simulink model "s_dbip"  (Simulink 7.7)
settings: Solver=ode1  StartTime=0.0  StopTime=100  FixedStep=0.001  RelTol=1e-3
values from neighbouring files (symbols this model uses):
  A = [0 0 0 1 0 0 ... (first row only)    [DBIP_ABCD_eqns.m]
  B = Kg * kt * B / Rm    [DBIP_ABCD_eqns.m]    (also in Symbolic_EL_Calculations.m = [1;0])
  C = eye(6,6)    [DBIP_ABCD_eqns.m]    (also in Symbolic_EL_Calculations.m = [0 theta2dot*sin(theta1 - theta2))
  D = zeros(6,1)    [DBIP_ABCD_eqns.m]
  X0 = [-5, 1, -0.5, 0, 0, 0] * pi / 180    [setup_dbip.m]
undefined symbols (not defined in the file or in its folder): k
libraries: simulink_extras x5
settings Model: Creator=MLevis  LastModifiedBy=MLevis  ExtModeTrigDuration=10000  ExtModeArmWhenConnect=off  BufferReuse=off
settings SolverCC: PositivePriorityOrder=on
settings OptimizationCC: BooleanDataType=off  InlineInvariantSignals=on  OptimizeBlockIOStorage=off  BufferReuse=off  ExpressionFolding=off  LocalBlockOutputs=off  InitFltsAndDblsToZero=on
settings DebuggingCC: SaveWithParameterizedLinksMsg=none  SignalResolutionControl=TryResolveAllWithWarning  SolverPrmCheckMsg=none  MultiTaskDSMMsg=warning  MultiTaskCondExecSysMsg=none  StrictBusMsg=None
settings RTWCC: SystemTargetFile=quarc_windows.tlc  TemplateMakefile=quarc_default_tmf  Description=QuaRC Win32 Target  ProcessScript=quarc_windows_make_rtw_hook  IncludeERTFirstTime=on
settings STFCustomTargetCC: TargetFcnLib=ansi_tfl_tmw.mat  TargetPreCompLibLocation=C:\PROGRA~3\QUARC\lib\2011a\windows\release  FunctionExecutionProfile=off  GeneratePreprocessorConditionals=Disable all  SystemTargetFile=quarc_windows.tlc
settings GRTTargetCC: TargetFcnLib=ansi_tfl_tmw.mat  TargetPreCompLibLocation=C:\PROGRA~3\QUARC\lib\2011a\windows\release  ParMdlRefBuildCompliant=off  CompOptLevelCompliant=off  MatFileLogging=off  ExtMode=on  ExtModeMexFile=quarc_comm

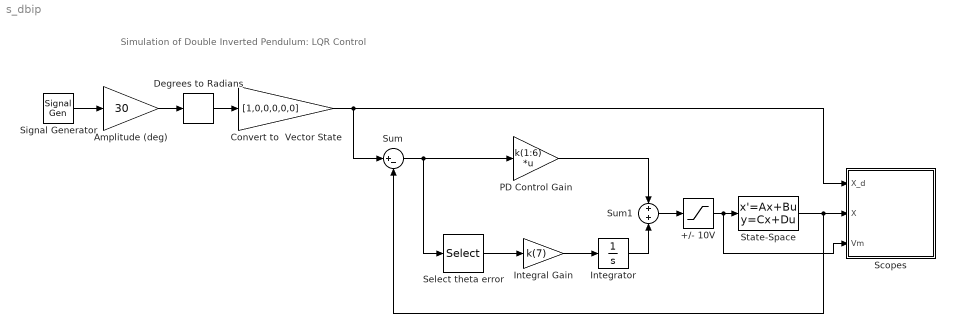
== system s_dbip ==
  note: Simulation of Double Inverted Pendulum: LQR Control
  +/- 10V : Saturate  UpperLimit=10  LowerLimit=-10
  Amplitude (deg) : Gain  Gain=30  SaturateOnIntegerOverflow=on  OutDataTypeStr=Inherit: Same as input  ParamDataTypeStr=Inherit: Same as input
  Convert to  Vector State : Gain  Gain=[1,0,0,0,0,0]
  Degrees to Radians : simulink_extras/Transformations/Degrees to Radians  SystemSampleTime=-1
  Integral Gain : Gain  Gain=k(7)
  Integrator : Integrator
  PD Control Gain : Gain  Gain=k(1:6)  Multiplication=Matrix(K*u)  SaturateOnIntegerOverflow=on  OutDataTypeStr=Inherit: Same as input  ParamDataTypeStr=Inherit: Same as input
  Scopes : Subsystem
  Select theta error : Selector  InputPortWidth=6  IndexOptions=Index vector (dialog)  Indices=1  OutputSizes=1
  Signal Generator : SignalGenerator  WaveForm=square  Frequency=0.02
  State-Space : StateSpace  A=A  B=B  C=C  D=D  X0=X0
  Sum : Sum  Inputs=|+-
  Sum1 : Sum
  wires:
  Signal Generator/1 -> Amplitude (deg)/1
  Amplitude (deg)/1 -> Degrees to Radians/1
  Degrees to Radians/1 -> Convert to  Vector State/1
  Convert to  Vector State/1 -> Sum/1, Scopes/1(X_d)
  Sum/1 -> PD Control Gain/1, Select theta error/1
  Sum1/1 -> +/- 10V/1
  Integral Gain/1 -> Integrator/1
  Select theta error/1 -> Integral Gain/1
  Integrator/1 -> Sum1/2
  PD Control Gain/1 -> Sum1/1
  State-Space/1 -> Scopes/2(X), Sum/2
  +/- 10V/1 -> State-Space/1, Scopes/3(Vm)

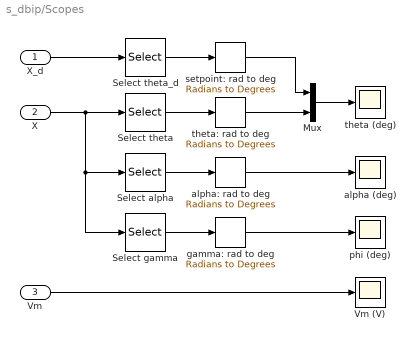
== system s_dbip/Scopes ==
  X_d : Inport
  X : Inport  Port=2
  Vm : Inport  Port=3
  Mux : Mux  Inputs=2
  Select alpha : Selector  InputPortWidth=6  IndexOptions=Index vector (dialog)  Indices=2  OutputSizes=1
  Select gamma : Selector  InputPortWidth=6  IndexOptions=Index vector (dialog)  Indices=3  OutputSizes=1
  Select theta : Selector  InputPortWidth=6  IndexOptions=Index vector (dialog)  Indices=1  OutputSizes=1
  Select theta_d : Selector  InputPortWidth=6  IndexOptions=Index vector (dialog)  Indices=1  OutputSizes=1
  Vm (V) : Scope
      settings: TickLabels=on  YMin=-4.5  YMax=4.5  SaveName=data_vm  DataFormat=Array
  alpha (deg) : Scope
      settings: SaveName=data_alpha  DataFormat=Array
  alpha: rad to deg : simulink_extras/Transformations/Radians to Degrees  SystemSampleTime=-1
  gamma: rad to deg : simulink_extras/Transformations/Radians to Degrees  SystemSampleTime=-1
  phi (deg) : Scope
      settings: SaveName=data_phi  DataFormat=Array
  setpoint: rad to deg : simulink_extras/Transformations/Radians to Degrees  SystemSampleTime=-1
  theta (deg) : Scope
      settings: YMin=-100  YMax=100  SaveName=data_theta  DataFormat=Array
  theta: rad to deg : simulink_extras/Transformations/Radians to Degrees  SystemSampleTime=-1
  wires:
  X/1 -> Select theta/1, Select alpha/1, Select gamma/1
  alpha: rad to deg/1 -> alpha (deg)/1
  gamma: rad to deg/1 -> phi (deg)/1
  Select theta/1 -> theta: rad to deg/1
  Select alpha/1 -> alpha: rad to deg/1
  Select gamma/1 -> gamma: rad to deg/1
  theta: rad to deg/1 -> Mux/2
  Mux/1 -> theta (deg)/1
  X_d/1 -> Select theta_d/1
  setpoint: rad to deg/1 -> Mux/1
  Select theta_d/1 -> setpoint: rad to deg/1
  Vm/1 -> Vm (V)/1
